simulink model "modelzbiornikow2"  (R2015a)
settings: Solver=ode3  SolverMode=SingleTasking  StartTime=0.0  StopTime=1000  FixedStep=0.01  RelTol=1e-3
values from neighbouring files (symbols this model uses):
  A = [-a1*C1*h1^(a1-1)/(a*w) 0 0;a1*C1*h1^(a1-1)/S1 -a2*C2*h2^(a2-1)/S1 0;0 a2*C2*h2^(a2-1)/S2 -a3*C3*h3^(a3-1)/S2]    [linearyzacja.m]
  a = 35    [linearyzacja.m]
  B = [1/(a*w); 0; 0]    [linearyzacja.m]
  b = 37    [linearyzacja.m]
  C = eye(3)    [linearyzacja.m]
  c = 10    [linearyzacja.m]
  D = [0; 0; 0]    [linearyzacja.m]
  h2max = 35    [linearyzacja.m]
  R = 36.4    [linearyzacja.m]
  w = 5    [linearyzacja.m]
undefined symbols (not defined in the file or in its folder): a1, a2, a3, C1, C2, C3
libraries: simulink x3
settings Model: Creator=Ziger  LastModifiedBy=Student
settings OptimizationCC: BlockReduction=off  BooleanDataType=off
settings DebuggingCC: SaveWithParameterizedLinksMsg=none  UnderspecifiedInitializationDetection=Classic  MergeDetectMultiDrivingBlocksExec=none  SignalResolutionControl=TryResolveAllWithWarning  MaxConsecutiveZCsMsg=none
settings HardwareCC: TargetUnknown=on

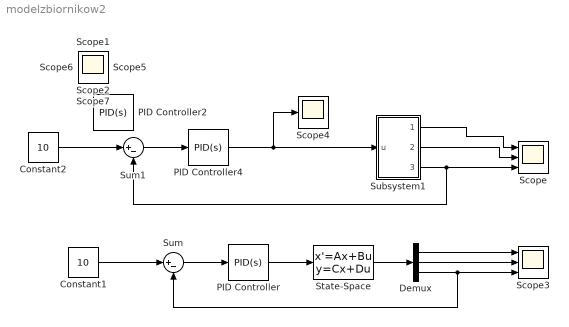
== system modelzbiornikow2 ==
  Constant1 : Constant  Value=10
  Constant2 : Constant  Value=10
  Demux : Demux  Outputs=3
  PID Controller : simulink/Continuous/PID Controller  Controller=PID  TimeDomain=Continuous-time  SampleTime=-1  IntegratorMethod=Forward Euler  FilterMethod=Forward Euler  Form=Parallel  UseFilter=on  ControllerParametersSource=internal  P=98.3041863849689  I=0.788822216002151  D=3008.19695181474  N=22.121248845653  InitialConditionSource=internal  InitialConditionForIntegrator=0  InitialConditionForFilter=0  ExternalReset=none  LimitOutput=on  UpperSaturationLimit=160  LowerSaturationLimit=0  LinearizeAsGain=off  AntiWindupMode=none  Kb=1  TrackingMode=off  Kt=1  PParamMin=[]  PParamMax=[]  IParamMin=[]  IParamMax=[]  DParamMin=[]  DParamMax=[]  NParamMin=[]  NParamMax=[]  KbParamMin=[]  KbParamMax=[]  KtParamMin=[]  KtParamMax=[]  POutMin=[]  POutMax=[]  IOutMin=[]  IOutMax=[]  DOutMin=[]  DOutMax=[]  NOutMin=[]  NOutMax=[]  KbOutMin=[]  KbOutMax=[]  KtOutMin=[]  KtOutMax=[]  IntegratorOutMin=[]  IntegratorOutMax=[]  FilterOutMin=[]  FilterOutMax=[]  SumOutMin=[]  SumOutMax=[]  SumI1OutMin=[]  SumI1OutMax=[]  SumI2OutMin=[]  SumI2OutMax=[]  SumI3OutMin=[]  SumI3OutMax=[]  SumDOutMin=[]  SumDOutMax=[]  SaturationOutMin=[]  SaturationOutMax=[]  IntegratorContinuousStateAttributes=''  IntegratorStateMustResolveToSignalObject=off  IntegratorRTWStateStorageClass=Auto  FilterContinuousStateAttributes=''  FilterStateMustResolveToSignalObject=off  FilterRTWStateStorageClass=Auto  DifferentiatorICPrevScaledInput=0  DifferentiatorOutMin=[]  DifferentiatorOutMax=[]
  PID Controller2 : simulink/Continuous/PID Controller  Controller=PID  TimeDomain=Continuous-time  SampleTime=-1  IntegratorMethod=Forward Euler  FilterMethod=Forward Euler  Form=Parallel  UseFilter=on  ControllerParametersSource=internal  P=17.7238005479891  I=0.157084159117056  D=493.15759754614  N=6.68051035088709  InitialConditionSource=internal  InitialConditionForIntegrator=0  InitialConditionForFilter=0  ExternalReset=none  LimitOutput=on  UpperSaturationLimit=160  LowerSaturationLimit=0  LinearizeAsGain=off  AntiWindupMode=none  Kb=1  TrackingMode=off  Kt=1  PParamMin=[]  PParamMax=[]  IParamMin=[]  IParamMax=[]  DParamMin=[]  DParamMax=[]  NParamMin=[]  NParamMax=[]  KbParamMin=[]  KbParamMax=[]  KtParamMin=[]  KtParamMax=[]  POutMin=[]  POutMax=[]  IOutMin=[]  IOutMax=[]  DOutMin=[]  DOutMax=[]  NOutMin=[]  NOutMax=[]  KbOutMin=[]  KbOutMax=[]  KtOutMin=[]  KtOutMax=[]  IntegratorOutMin=[]  IntegratorOutMax=[]  FilterOutMin=[]  FilterOutMax=[]  SumOutMin=[]  SumOutMax=[]  SumI1OutMin=[]  SumI1OutMax=[]  SumI2OutMin=[]  SumI2OutMax=[]  SumI3OutMin=[]  SumI3OutMax=[]  SumDOutMin=[]  SumDOutMax=[]  SaturationOutMin=[]  SaturationOutMax=[]  IntegratorContinuousStateAttributes=''  IntegratorStateMustResolveToSignalObject=off  IntegratorRTWStateStorageClass=Auto  FilterContinuousStateAttributes=''  FilterStateMustResolveToSignalObject=off  FilterRTWStateStorageClass=Auto  DifferentiatorICPrevScaledInput=0  DifferentiatorOutMin=[]  DifferentiatorOutMax=[]
  PID Controller4 : simulink/Continuous/PID Controller  Controller=PID  TimeDomain=Continuous-time  SampleTime=-1  IntegratorMethod=Forward Euler  FilterMethod=Forward Euler  Form=Parallel  UseFilter=on  ControllerParametersSource=internal  P=72.0668134198184  I=0.505184059209354  D=2505.73667524144  N=19.9072311343087  InitialConditionSource=internal  InitialConditionForIntegrator=0  InitialConditionForFilter=0  ExternalReset=none  LimitOutput=off  UpperSaturationLimit=160  LowerSaturationLimit=0  LinearizeAsGain=off  AntiWindupMode=none  Kb=1  TrackingMode=off  Kt=1  PParamMin=[]  PParamMax=[]  IParamMin=[]  IParamMax=[]  DParamMin=[]  DParamMax=[]  NParamMin=[]  NParamMax=[]  KbParamMin=[]  KbParamMax=[]  KtParamMin=[]  KtParamMax=[]  POutMin=[]  POutMax=[]  IOutMin=[]  IOutMax=[]  DOutMin=[]  DOutMax=[]  NOutMin=[]  NOutMax=[]  KbOutMin=[]  KbOutMax=[]  KtOutMin=[]  KtOutMax=[]  IntegratorOutMin=[]  IntegratorOutMax=[]  FilterOutMin=[]  FilterOutMax=[]  SumOutMin=[]  SumOutMax=[]  SumI1OutMin=[]  SumI1OutMax=[]  SumI2OutMin=[]  SumI2OutMax=[]  SumI3OutMin=[]  SumI3OutMax=[]  SumDOutMin=[]  SumDOutMax=[]  SaturationOutMin=[]  SaturationOutMax=[]  IntegratorContinuousStateAttributes=''  IntegratorStateMustResolveToSignalObject=off  IntegratorRTWStateStorageClass=Auto  FilterContinuousStateAttributes=''  FilterStateMustResolveToSignalObject=off  FilterRTWStateStorageClass=Auto  DifferentiatorICPrevScaledInput=0  DifferentiatorOutMin=[]  DifferentiatorOutMax=[]
  Scope : Scope  NumInputPorts=3
      settings: YMin=0~0~0  YMax=10~5.5~11  SaveName=zbiorniki
  Scope3 : Scope  NumInputPorts=3
      settings: YMin=0~0~0.095  YMax=1e-44~1.1e-41~0.105  SaveName=zbiorniki1
  Scope{1..2,4..7} (6 alike) : Scope
      Scope4 settings: YMin=0  YMax=1e-44  SaveName=zbiorniki2
      Scope5 settings: SaveName=ScopeData2
      Scope6 settings: SaveName=ScopeData3
      Scope7 settings: SaveName=ScopeData4
  State-Space : StateSpace  A=A  B=B  C=C  D=D  X0=0
  Subsystem1 : Subsystem
  Sum : Sum  Inputs=|+-
  Sum1 : Sum  Inputs=|+-
  wires:
  Subsystem1/1(h1out) -> Scope/1
  Subsystem1/2("h2out ") -> Scope/2
  Demux/3 -> Sum/2, Scope3/3
  Demux/2 -> Scope3/2
  Demux/1 -> Scope3/1
  State-Space/1 -> Demux/1
  PID Controller/1 -> State-Space/1
  Sum/1 -> PID Controller/1
  Constant1/1 -> Sum/1
  Subsystem1/3("h3out ") -> Sum1/2, Scope/3
  PID Controller4/1 -> Scope4/1, Subsystem1/1(u)
  Sum1/1 -> PID Controller4/1
  Constant2/1 -> Sum1/1

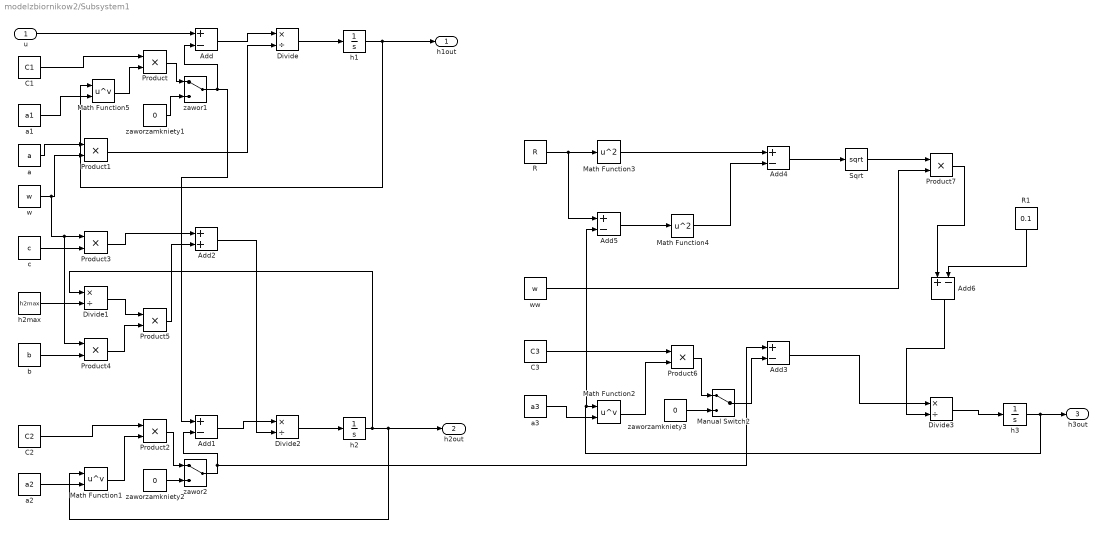
== system modelzbiornikow2/Subsystem1 ==
  u : Inport
  Add{,1,3..6} (6 alike) : Sum  Inputs=+-
  Add2 : Sum
  C1 : Constant  Value=C1
  C2 : Constant  Value=C2
  C3 : Constant  Value=C3
  Divide{,1..3} (4 alike) : Product  Inputs=*/
  Manual Switch2 : ManualSwitch
  Math Function1 : Math  Operator=pow  SaturateOnIntegerOverflow=on
  Math Function2 : Math  Operator=pow  SaturateOnIntegerOverflow=on
  Math Function3 : Math  Operator=square  SaturateOnIntegerOverflow=on
  Math Function4 : Math  Operator=square  SaturateOnIntegerOverflow=on
  Math Function5 : Math  Operator=pow  SaturateOnIntegerOverflow=on
  Product{,1..7} (8 alike) : Product
  R : Constant  Value=R
  R1 : Constant  Value=0.1
  Sqrt : Sqrt  SaturateOnIntegerOverflow=on
  a : Constant  Value=a
  a1 : Constant  Value=a1
  a2 : Constant  Value=a2
  a3 : Constant  Value=a3
  b : Constant  Value=b
  c : Constant  Value=c
  h1 : Integrator  LimitOutput=on  UpperSaturationLimit=35  LowerSaturationLimit=0
  h2 : Integrator  LimitOutput=on  UpperSaturationLimit=35  LowerSaturationLimit=0
  h2max : Constant  Value=h2max
  h3 : Integrator  InitialCondition=0.1  LimitOutput=on  UpperSaturationLimit=35  LowerSaturationLimit=0
  w : Constant  Value=w
  ww : Constant  Value=w
  "zawor1 " : ManualSwitch
  "zawor2 " : ManualSwitch
  zaworzamkniety1 : Constant  Value=0
  zaworzamkniety2 : Constant  Value=0
  zaworzamkniety3 : Constant  Value=0
  h1out : Outport
  "h2out " : Outport  Port=2
  "h3out " : Outport  Port=3
  wires:
  h1/1 -> Math Function5/1, h1out/1
  h2/1 -> Divide1/1, "h2out "/1, Math Function1/1
  Math Function1/1 -> Product2/2
  u/1 -> Add/1
  Add/1 -> Divide/1
  Product/1 -> "zawor1 "/1
  C1/1 -> Product/1
  a/1 -> Product1/1
  Product4/1 -> Product5/2
  Product1/1 -> Divide/2
  h2max/1 -> Divide1/2
  C2/1 -> Product2/1
  w/1 -> Product4/1, Product3/1, Product1/2
  Divide2/1 -> h2/1
  Add2/1 -> Divide2/2
  Divide1/1 -> Product5/1
  a2/1 -> Math Function1/2
  Product5/1 -> Add2/2
  Add3/1 -> Divide3/1
  R/1 -> Add5/1, Math Function3/1
  h3/1 -> "h3out "/1, Add5/2, Math Function2/1
  Math Function3/1 -> Add4/1
  Add4/1 -> Sqrt/1
  Divide3/1 -> h3/1
  Sqrt/1 -> Product7/1
  Math Function2/1 -> Product6/2
  b/1 -> Product4/2
  Add5/1 -> Math Function4/1
  a3/1 -> Math Function2/2
  Product3/1 -> Add2/1
  C3/1 -> Product6/1
  ww/1 -> Product7/2
  Math Function4/1 -> Add4/2
  Add1/1 -> Divide2/1
  c/1 -> Product3/2
  zaworzamkniety1/1 -> "zawor1 "/2
  "zawor1 "/1 -> Add1/1, Add/2
  Product2/1 -> "zawor2 "/1
  zaworzamkniety2/1 -> "zawor2 "/2
  "zawor2 "/1 -> Add3/1, Add1/2
  Product6/1 -> Manual Switch2/1
  zaworzamkniety3/1 -> Manual Switch2/2
  Manual Switch2/1 -> Add3/2
  Divide/1 -> h1/1
  a1/1 -> Math Function5/2
  Math Function5/1 -> Product/2
  Product7/1 -> Add6/1
  Add6/1 -> Divide3/2
  R1/1 -> Add6/2
